simulink model "planarPlotTestN1"  (R2024b)
settings: Solver=VariableStepAuto  StartTime=0.0  StopTime=10.0  RelTol=1e-3
model workspace (MAT data in the model file):
  Nn = Simulink.Parameter
  Nn.Value = 0.001
  Nn.Complexity = 'real'
  Nn.Dimensions = [1 1]
  Nn.DataType = 'auto'
  Sig = Simulink.Signal
  Sig.Dimensions = -1
  Sig.DimensionsMode = 'auto'
  Sig.Complexity = 'auto'
  Sig.SampleTime = -1
  Sig.SamplingMode = 'auto'
  Sig.DataType = 'auto'
  jointOmega = Simulink.Parameter
  jointOmega.Value = [0 0 0]
  jointOmega.Complexity = 'real'
  jointOmega.Dimensions = [1 3]
  jointOmega.DataType = 'auto'
  jointOmega1 = Simulink.Parameter
  jointOmega1.Value = -0.6
  jointOmega1.Complexity = 'real'
  jointOmega1.Dimensions = [1 1]
  jointOmega1.DataType = 'auto'
  jointOmega2 = Simulink.Parameter
  jointOmega2.Value = -0.3
  jointOmega2.Complexity = 'real'
  jointOmega2.Dimensions = [1 1]
  jointOmega2.DataType = 'auto'
  jointOmega3 = Simulink.Parameter
  jointOmega3.Value = 0
  jointOmega3.Complexity = 'real'
  jointOmega3.Dimensions = [1 1]
  jointOmega3.DataType = 'auto'
  jointTheta = Simulink.Parameter
  jointTheta.Value = 0
  jointTheta.Complexity = 'real'
  jointTheta.Dimensions = [1 1]
  jointTheta.DataType = 'auto'
  jointTheta.Min = -2.09439510239
  jointTheta.Max = 2.09439510239
  jointTheta1 = Simulink.Parameter
  jointTheta1.Value = -1
  jointTheta1.Complexity = 'real'
  jointTheta1.Dimensions = [1 1]
  jointTheta1.DataType = 'auto'
  jointTheta2 = Simulink.Parameter
  jointTheta2.Value = 1.2
  jointTheta2.Complexity = 'real'
  jointTheta2.Dimensions = [1 1]
  jointTheta2.DataType = 'auto'
  jointTheta3 = Simulink.Parameter
  jointTheta3.Value = -0.5
  jointTheta3.Complexity = 'real'
  jointTheta3.Dimensions = [1 1]
  jointTheta3.DataType = 'auto'
libraries: simulink x1
settings Model: Creator=vince  LastModifiedBy=vince

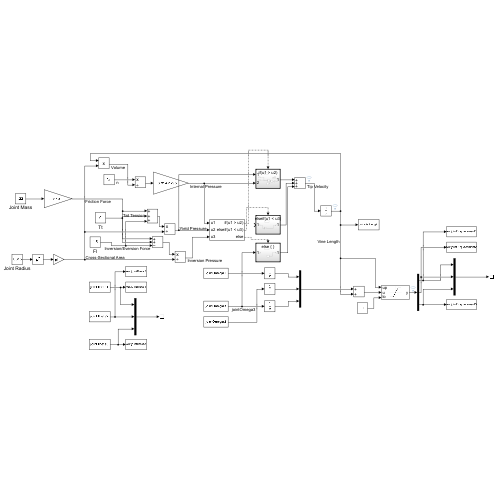
[thumbnail: Simulink's stored preview of the top-level diagram]
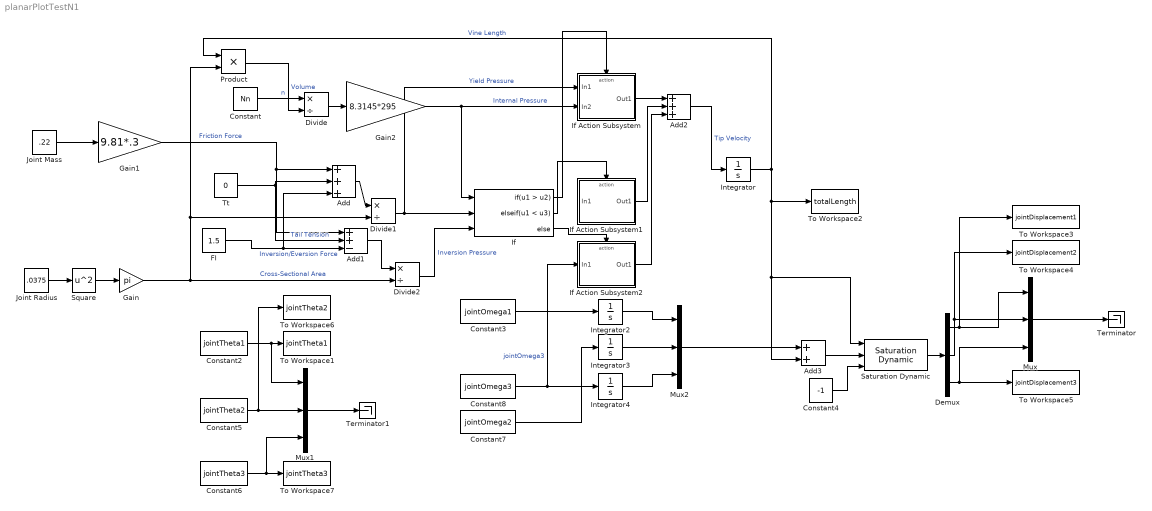
== system planarPlotTestN1 ==
  Add : Sum  Inputs=+++
  Add1 : Sum  Inputs=++-
  Add2 : Sum  Inputs=+++
  Add3 : Sum
  Constant : Constant  Value=Nn
  Constant2 : Constant  Value=jointTheta1
  Constant3 : Constant  Value=jointOmega1
  Constant4 : Constant  Value=-1
  Constant5 : Constant  Value=jointTheta2
  Constant6 : Constant  Value=jointTheta3
  Constant7 : Constant  Value=jointOmega2
  Constant8 : Constant  Value=jointOmega3
  Demux : Demux  Outputs=3
  Divide : Product  Inputs=*/
  Divide1 : Product  Inputs=*/
  Divide2 : Product  Inputs=*/
  FI : Constant  Value=1.5
  Gain : Gain  Gain=pi
  Gain1 : Gain  Gain=9.81*.3
  Gain2 : Gain  Gain=8.3145*295
  If : If  NumInputs=3  IfExpression=u1 > u2  ElseIfExpressions=u1 < u3
  If Action Subsystem : Subsystem  TreatAsAtomicUnit=on
  If Action Subsystem1 : Subsystem  TreatAsAtomicUnit=on
  If Action Subsystem2 : Subsystem  TreatAsAtomicUnit=on
  Integrator : Integrator  InitialCondition=1
  Integrator2 : Integrator  InitialCondition=-.9
  Integrator3 : Integrator  InitialCondition=-.6
  Integrator4 : Integrator  InitialCondition=-.3
  Joint Mass : Constant  Value=.22
  Joint Radius : Constant  Value=.0375
  Mux : Mux  Inputs=3
  Mux1 : Mux  Inputs=3
  Mux2 : Mux  Inputs=3
  Product : Product
  Saturation Dynamic : simulink/Discontinuities/Saturation Dynamic  OutMin=[]  OutMax=[]  OutDataTypeStr=Inherit: Same as second input  OutDataType=fixdt(1, 16)  OutScaling=2^-10  DoSatur=off
  Square : Math  Operator=square
  Terminator : Terminator
  Terminator1 : Terminator
  To Workspace1 : ToWorkspace  VariableName=jointTheta1  SaveFormat=Timeseries  SampleTime=-1
  To Workspace2 : ToWorkspace  VariableName=totalLength  SaveFormat=Timeseries  SampleTime=-1
  To Workspace3 : ToWorkspace  VariableName=jointDisplacement1  SaveFormat=Timeseries  SampleTime=-1
  To Workspace4 : ToWorkspace  VariableName=jointDisplacement2  SaveFormat=Timeseries  SampleTime=-1
  To Workspace5 : ToWorkspace  VariableName=jointDisplacement3  SaveFormat=Timeseries  SampleTime=-1
  To Workspace6 : ToWorkspace  VariableName=jointTheta2  SaveFormat=Timeseries  SampleTime=-1
  To Workspace7 : ToWorkspace  VariableName=jointTheta3  SaveFormat=Timeseries  SampleTime=-1
  Tt : Constant  Value=0
  wires:
  Constant/1 -> Divide/1  "n"
  Constant2/1 -> Mux1/1, To Workspace1/1
  Add3/1 -> Saturation Dynamic/2
  Constant3/1 -> Integrator2/1
  Joint Radius/1 -> Square/1
  Demux/2 -> To Workspace4/1, Mux/2
  Constant4/1 -> Saturation Dynamic/3
  Constant8/1 -> Integrator4/1, If Action Subsystem2/1(In1)  "jointOmega3"
  Constant6/1 -> Mux1/3, To Workspace7/1
  Constant7/1 -> Integrator3/1
  Constant5/1 -> Mux1/2, To Workspace6/1
  Square/1 -> Gain/1
  Divide/1 -> Gain2/1
  Joint Mass/1 -> Gain1/1
  Mux1/1 -> Terminator1/1
  Gain/1 -> Product/2, Divide1/2, Divide2/2  "Cross-Sectional Area"
  Mux2/1 -> Add3/1
  Product/1 -> Divide/2  "Volume"
  Gain1/1 -> Add1/1, Add/1  "Friction Force"
  Tt/1 -> Add/2, Add1/2  "Tail Tension"
  FI/1 -> Add1/3, Add/3  "Inversion/Eversion Force"
  Add/1 -> Divide1/1
  Demux/3 -> Mux/3, To Workspace5/1
  Add1/1 -> Divide2/1
  If/2 -> If Action Subsystem1/Action
  Gain2/1 -> If Action Subsystem/2(In2), If/1  "Internal Pressure"
  Divide2/1 -> If/3  "Inversion Pressure"
  Divide1/1 -> If Action Subsystem/1(In1), If/2  "Yield Pressure"
  If/3 -> If Action Subsystem2/Action
  If/1 -> If Action Subsystem/Action
  If Action Subsystem/1(Out1) -> Add2/1
  If Action Subsystem1/1(Out1) -> Add2/2
  If Action Subsystem2/1(Out1) -> Add2/3
  Mux/1 -> Terminator/1
  Integrator2/1 -> Mux2/1
  Integrator3/1 -> Mux2/2
  Integrator4/1 -> Mux2/3
  Add2/1 -> Integrator/1  "Tip Velocity"
  Integrator/1 -> Saturation Dynamic/1, Add3/2, To Workspace2/1, Product/1  "Vine Length"
  Saturation Dynamic/1 -> Demux/1
  Demux/1 -> To Workspace3/1, Mux/1

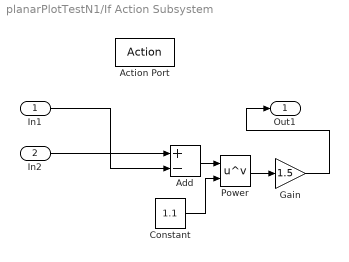
== system planarPlotTestN1/If Action Subsystem ==
  In1 : Inport
  In2 : Inport  Port=2
  Action Port : ActionPort  ActionPortLabel=if(u1 > u2)
  Add : Sum  Inputs=+-
  Constant : Constant  Value=1.1
  Gain : Gain  Gain=1.5
  Power : Math  Operator=pow
  Out1 : Outport
  wires:
  In2/1 -> Add/1
  In1/1 -> Add/2
  Add/1 -> Power/1
  Power/1 -> Gain/1
  Constant/1 -> Power/2
  Gain/1 -> Out1/1

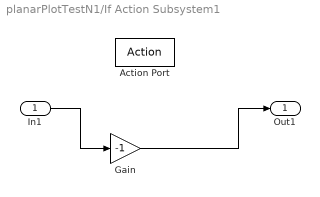
== system planarPlotTestN1/If Action Subsystem1 ==
  In1 : Inport
  Action Port : ActionPort  ActionPortLabel=elseif(u1 < u3)
  Gain : Gain  Gain=-1
  Out1 : Outport
  wires:
  Gain/1 -> Out1/1
  In1/1 -> Gain/1

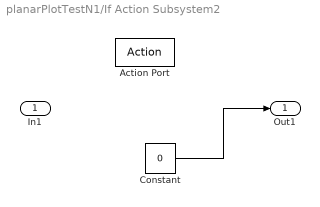
== system planarPlotTestN1/If Action Subsystem2 ==
  In1 : Inport
  Action Port : ActionPort  ActionPortLabel=else
  Constant : Constant  Value=0
  Out1 : Outport
  wires:
  Constant/1 -> Out1/1
